simulink model "Generic_sedan"  (R2023b)
settings: Solver=VariableStepAuto  StartTime=0.0  StopTime=26  FixedStep=0.001  MaxStep=0.01  RelTol=1e-4
InitFcn:
  | A = readmatrix(['data' filesep 'A.dat']);
  | B = readmatrix(['data' filesep 'B.dat']);
  | C = readmatrix(['data' filesep 'C.dat']);
  | D = readmatrix(['data' filesep 'D.dat']);
  | 
  | Z0 = readmatrix(['data' filesep 'Z0.dat']);
  | m = readmatrix(['data' filesep 'mass.dat']);
  | IG = readmatrix(['data' filesep 'IG.dat']);
  | 
  | z = readmatrix(['data' filesep 'z.dat']);
  | l = readmatrix(['data' filesep 'l.dat']);
  | fbf = readmatrix(['data' filesep 'brake.dat']);
libraries: simulink x10, matrix_library x2, slpidlib x1
(part 2 of 2)

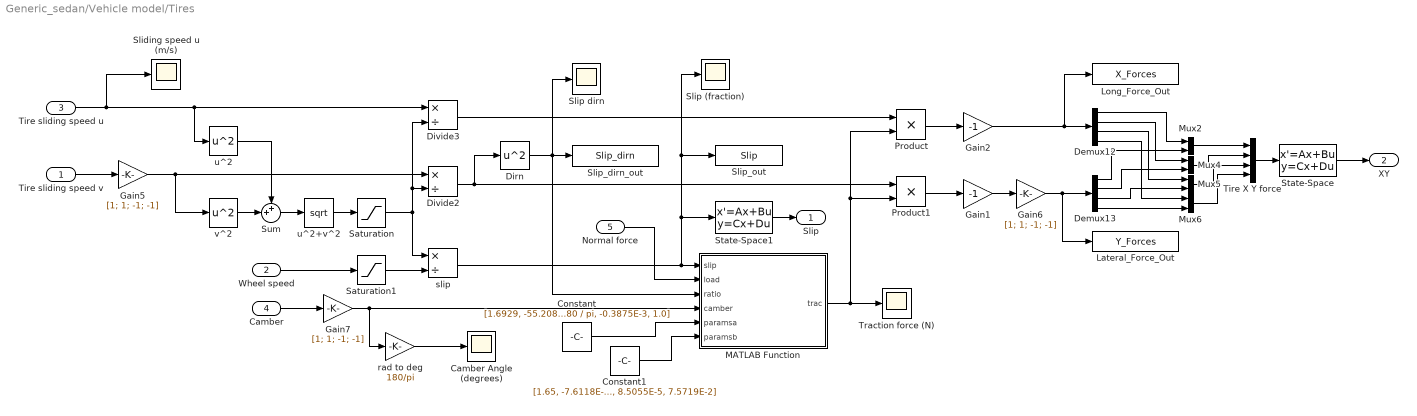
== system Generic_sedan/Vehicle model/Tires ==
  Tire sliding speed v : Inport
  Wheel speed : Inport  Port=2
  Tire sliding speed u : Inport  Port=3
  Camber : Inport  Port=4
  Normal force : Inport  Port=5
  Camber Angle (degrees) : Scope
  Constant : Constant  Value=[1.6929, -55.2084E-6, 1.27128, 1601.8 * 180 / pi, 6494.6, 4.7966E-3 * 180 / pi, -0.3875E-3, 1.0]
  Constant1 : Constant  Value=[1.65, -7.6118E-6, 1.1226, -7.36E-7, 14.482, -7.6614E-5, -3.86E-9, 8.5055E-5, 7.5719E-2]
  Demux12 : Demux
  Demux13 : Demux
  Dirn : Math  Operator=square
  Divide2 : Product  Inputs=*/
  Divide3 : Product  Inputs=*/
  Gain1 : Gain  Gain=-1
  Gain2 : Gain  Gain=-1
  Gain5 : Gain  Gain=[1; 1; -1; -1]
  Gain6 : Gain  Gain=[1; 1; -1; -1]
  Gain7 : Gain  Gain=[1; 1; -1; -1]
  Lateral_Force_Out : ToWorkspace  VariableName=Y_Forces  SaveFormat=Timeseries  SampleTime=-1
      settings: Decimation=3
  Long_Force_Out : ToWorkspace  VariableName=X_Forces  SaveFormat=Timeseries  SampleTime=-1
      settings: Decimation=3
  MATLAB Function : MATLAB Function  TreatAsAtomicUnit=on
  Mux{2,4..6} (4 alike) : Mux  Inputs=2
  Product : Product
  Product1 : Product
  Saturation : Saturate  UpperLimit=Inf  LowerLimit=1e-9
  Saturation1 : Saturate  UpperLimit=Inf  LowerLimit=0.1
  Sliding speed u (m/s) : Scope
  Slip (fraction) : Scope
  Slip dirn : Scope
  Slip_dirn_out : ToWorkspace  VariableName=Slip_dirn  SaveFormat=Timeseries  SampleTime=-1
      settings: Decimation=3
  Slip_out : ToWorkspace  VariableName=Slip  SaveFormat=Timeseries  SampleTime=-1
      settings: Decimation=3
  State-Space : StateSpace  A=-100 *eye(8)  B=100*eye(8)  C=eye(8)  D=zeros(8,8)  InitialCondition=0
  State-Space1 : StateSpace  A=-100 *eye(4)  B=100*eye(4)  C=eye(4)  D=zeros(4,4)  InitialCondition=0
  Sum : Sum  Inputs=++|
  Tire X Y force : Mux
  Traction force (N) : Scope
  rad to deg : Gain  Gain=180/pi
  slip : Product  Inputs=*/
  u^2 : Math  Operator=square
  u^2+v^2 : Sqrt
  v^2 : Math  Operator=square
  Slip : Outport
  XY : Outport  Port=2
  wires:
  Gain5/1 -> v^2/1, Divide2/1
  Tire sliding speed u/1 -> u^2/1, Divide3/1, Sliding speed u (m/s)/1
  Sum/1 -> u^2+v^2/1
  v^2/1 -> Sum/2
  u^2/1 -> Sum/1
  Wheel speed/1 -> Saturation1/1
  Normal force/1 -> MATLAB Function/2(load)
  Camber/1 -> Gain7/1
  MATLAB Function/1(trac) -> Traction force (N)/1, Product1/2, Product/2
  Product1/1 -> Gain1/1
  Constant/1 -> MATLAB Function/5(paramsa)
  Constant1/1 -> MATLAB Function/6(paramsb)
  Gain1/1 -> Gain6/1
  Product/1 -> Gain2/1
  Divide3/1 -> Product/1
  slip/1 -> MATLAB Function/1(slip), State-Space1/1, Slip (fraction)/1, Slip_out/1
  Dirn/1 -> Slip_dirn_out/1, Slip dirn/1, MATLAB Function/3(ratio)
  Tire sliding speed v/1 -> Gain5/1
  Demux12/4 -> Mux6/1
  Mux2/1 -> Tire X Y force/1
  Mux5/1 -> Tire X Y force/3
  Demux13/3 -> Mux5/2
  Demux13/1 -> Mux2/2
  Demux13/4 -> Mux6/2
  Demux12/1 -> Mux2/1
  Demux12/2 -> Mux4/1
  Mux4/1 -> Tire X Y force/2
  Gain6/1 -> Lateral_Force_Out/1, Demux13/1
  Gain2/1 -> Long_Force_Out/1, Demux12/1
  Demux13/2 -> Mux4/2
  Mux6/1 -> Tire X Y force/4
  Demux12/3 -> Mux5/1
  rad to deg/1 -> Camber Angle (degrees)/1
  Gain7/1 -> MATLAB Function/4(camber), rad to deg/1
  Saturation/1 -> slip/1, Divide3/2, Divide2/2
  Saturation1/1 -> slip/2
  u^2+v^2/1 -> Saturation/1
  Divide2/1 -> Product1/1, Dirn/1
  Tire X Y force/1 -> State-Space/1
  State-Space1/1 -> Slip/1
  State-Space/1 -> XY/1

== system Generic_sedan/Vehicle model/Traction cotrol ==
  Slip : Inport
  Demux2 : Demux
  Force cut : Lookup_n-D  NumberOfTableDimensions=1  BreakpointsForDimension1=[0,0.2,0.5,1]  Table=[1,1,0,0]  InternalRulePriority=Speed  RndMeth=Simplest
  Gain8 : Gain  Gain=0.5
  Mux1 : Mux  Inputs=2
  Sum1 : Sum  Inputs=|++
  Sum2 : Sum  Inputs=|++
  Limiter : Outport
  wires:
  Demux2/1 -> Sum1/1
  Sum2/1 -> Mux1/2
  Sum1/1 -> Mux1/1
  Demux2/4 -> Sum2/2
  Demux2/3 -> Sum1/2
  Gain8/1 -> Force cut/1
  Mux1/1 -> Gain8/1
  Demux2/2 -> Sum2/1
  Slip/1 -> Demux2/1
  Force cut/1 -> Limiter/1

== system Generic_sedan/Steering/FMVSS 126/Triggered Subsystem1 ==
  Trigger : TriggerPort  VariantControl=(inherit)
  Constant : Constant
  Out1 : Outport  InitialOutput=0
  wires:
  Constant/1 -> Out1/1

== system Generic_sedan/Steering/Steer - sweep/Triggered Subsystem ==
  In1 : Inport
  Trigger : TriggerPort  VariantControl=(inherit)
  A : Outport
  wires:
  In1/1 -> A/1

== matlab function Generic_sedan/Vehicle model/Tires/MATLAB Function ==
  data: slip input; trac output; load input; ratio input; camber input; paramsa input; paramsb input
function trac = tire_comb(slip, load, ratio, camber, paramsa, paramsb)

    one_minus_ratio = 1.0 - ratio;

    C = paramsa(1) * ratio + paramsb(1) * one_minus_ratio;
    mu_p = (paramsa(2) * ratio + paramsb(2) * one_minus_ratio) .* load + (paramsa(3) * ratio + paramsb(3) * one_minus_ratio);
    D = mu_p .* load;

    Ea = paramsa(7) * load + paramsa(8);
    Eb = paramsb(7) * load .^ 2 + paramsb(8) * load + paramsb(9);
    E = ratio .* Ea + one_minus_ratio .* Eb;

    Ba = paramsa(4) * sin(2 * atan(load / paramsa(5))) .* (1.0 - paramsa(6) * abs(camber)) ./ C ./ D;
    Bb = (paramsb(4) * load .^ 2 + paramsb(5) * load) .* exp(-paramsb(6) * load) ./ C ./ D;
    B = ratio .* Ba + one_minus_ratio .* Bb;

    trac = D .* sin(C .* atan(B .* (1.0 - E) .* slip + E .* atan(B .* slip)));
